simulink model "q2i"  (R2018a)
settings: Solver=FixedStepAuto  StartTime=0.0  StopTime=10.0  FixedStep=0.00001  RelTol=1e-3
libraries: simulink x1
settings Model: Creator=hp  LastModifiedBy=hp

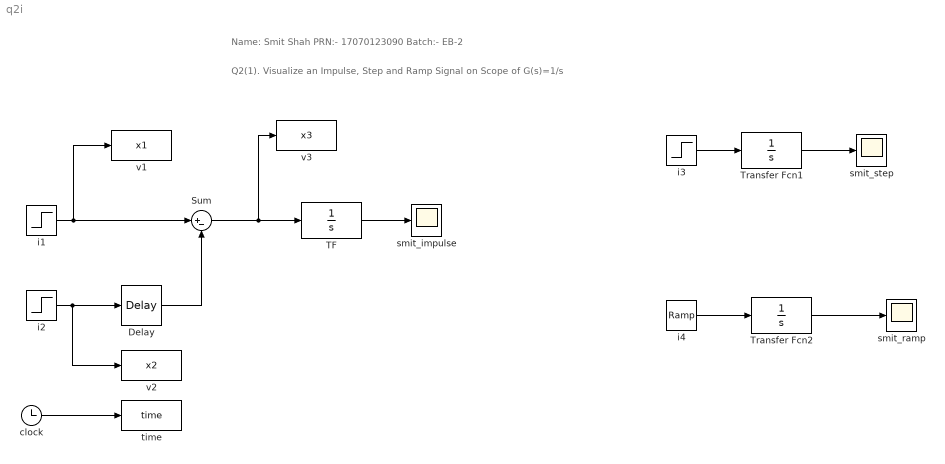
== system q2i ==
  note: Name: Smit Shah PRN:- 17070123090 Batch:- EB-2
  note: Q2(1). Visualize an Impulse, Step and Ramp Signal on Scope of G(s)=1/s
  Delay : TransportDelay  DelayTime=0.00001
  Sum : Sum  Inputs=|+-
  TF : TransferFcn  Denominator=[1 0]
  Transfer Fcn1 : TransferFcn  Denominator=[1 0]
  Transfer Fcn2 : TransferFcn  Denominator=[1 0]
  clock : Clock
  i1 : Step  Time=0  SampleTime=0
  i2 : Step  Time=0  After=2  SampleTime=0
  i3 : Step  Time=0  SampleTime=0
  i4 : simulink/Sources/Ramp  slope=1  start=0  InitialOutput=0
  smit_impulse : Scope
  smit_ramp : Scope
  smit_step : Scope
  time : ToWorkspace  VariableName=time  SampleTime=-1
  v1 : ToWorkspace  VariableName=x1  SampleTime=-1
  v2 : ToWorkspace  VariableName=x2  SampleTime=-1
  v3 : ToWorkspace  VariableName=x3  SampleTime=-1
  wires:
  i1/1 -> Sum/1, v1/1
  i2/1 -> v2/1, Delay/1
  clock/1 -> time/1
  Delay/1 -> Sum/2
  Sum/1 -> TF/1, v3/1
  TF/1 -> smit_impulse/1
  Transfer Fcn2/1 -> smit_ramp/1
  i3/1 -> Transfer Fcn1/1
  i4/1 -> Transfer Fcn2/1
  Transfer Fcn1/1 -> smit_step/1
